simulink model "VehicleDynamics3D"  (R2019b)
settings: Solver=ode15s  StartTime=0.0  StopTime=StopTime  FixedStep=.001  MaxStep=maxStep  RelTol=relTol  AbsTol=absTol  EnableMultiTasking=on
PreLoadFcn:
  | VehicleDynamicsInitialization
model workspace: external: MATLAB File sm_suspension_templates_params.m (data not in the file)
values from neighbouring files (symbols this model uses):
  followerCameraX = 7.5    [VehicleDynamicsInitialization.m]
  followerCameraZ = 3    [VehicleDynamicsInitialization.m]
  frontCameraX = -1.75    [VehicleDynamicsInitialization.m]
  frontCameraZ = 0.35    [VehicleDynamicsInitialization.m]
  isoCameraAimX = (1/2)*wheelbase    (= 0.75)    [VehicleDynamicsInitialization.m]
  isoCameraX = -3.1    [VehicleDynamicsInitialization.m]
  isoCameraY = 3.5    [VehicleDynamicsInitialization.m]
  isoCameraZ = 1.5    [VehicleDynamicsInitialization.m]
  Load = 200    [VehicleDynamicsInitialization.m]
  maxSteeringDisplacement = 10    [VehicleDynamicsInitialization.m]
  minSteeringDisplacement = -10    [VehicleDynamicsInitialization.m]
  SetPaceSampleTime = 0.1    [VehicleDynamicsInitialization.m]
  steeringInput = 0    [VehicleDynamicsInitialization.m]
  vehicleSpeed_kph = 0    [VehicleDynamicsInitialization.m]
  wheelbase = 1.5    [VehicleDynamicsInitialization.m]
undefined symbols (not defined in the file or in its folder): dwb, Floor, sigbuilder_block, wheel, X, Y, Z
libraries: sm_lib x195, sm_suspension_templates_lib x34, nesl_utility x15, Contact_Forces_Lib x4, simulink x2, fl_ps_legacy_lib x1, aerolibanimutils x1
(part 1 of 8)
CloseFcn:
  | clear simlog_sm_suspension_templates
Description:
  | Independent Suspension System Templates
  | 
  | Copyright 2016-2017 The MathWorks, Inc.
settings Model: Creator=MathWorks  LastModifiedBy=adityaaaap
settings SolverCC: AutoScaleAbsTol=off  ZeroCrossAlgorithm=Adaptive
settings DataIOCC: SaveFormat=Array  SaveOutput=off  ReturnWorkspaceOutputsName=FrameCopy_spidata
settings OptimizationCC: ExpressionDepthLimit=2147483647  LifeSpan=inf
settings DebuggingCC: UnderspecifiedInitializationDetection=Classic  MergeDetectMultiDrivingBlocksExec=none  MaskedZcDiagnostic=none  IgnoredZcDiagnostic=none  AllowSymbolicDim=off  StateNameClashWarn=warning  SFUnexpectedBacktrackingDiag=warning  SFNoUnconditionalDefaultTransitionDiag=warning  SFExecutionAtInitializationDiag=none  ArithmeticOperatorsInVariantConditions=warning
settings HardwareCC: ProdBitPerPointer=32  ProdBitPerSizeT=32  ProdBitPerPtrDiffT=32  ProdLargestAtomicFloat=None  ProdIntDivRoundTo=Undefined  ProdEndianess=Unspecified  ProdWordSize=32  ProdHWDeviceType=32-bit Generic
settings ModelReferenceCC: PropagateSignalLabelsOutOfModel=off
settings SFSimCC: SimUseLocalCustomCode=off  SimBuildMode=sf_make  CustomCodeUndefinedFunction=UseInterfaceOnly
settings RTWCC: RTWUseLocalCustomCode=off
settings CodeAppCC: StateflowObjectComments=on
settings GRTTargetCC: TargetLangStandard=C89/C90 (ANSI)  GeneratePreprocessorConditionals=Disable all
settings ConfigComp: CovScope=ReferencedModels  CovIncludeTopModel=off  CovMetricSettings=dw  CovHtmlReporting=on  CovSaveCumulativeToWorkspaceVar=on  CovSaveSingleToWorkspaceVar=on  CovExternalEMLEnable=off  CovSFcnEnable=off
settings SimscapeCC: SimscapeNormalizeSystem=off  SimscapeLogSimulationStatistics=on  SimscapeLogLimitData=off  SimscapeLogDataHistory=10000
settings ConfigurationSet: Description=SimMechanics 2G
settings DiagnosticsConfigSet: SimMechanicsUnconnectedFramePorts=none  SimMechanicsRigidlyBoundBlock=none  SimMechanicsUnsatisfiedHighPriorityTargets=none
settings ExplorerConfigSet: InternalSimMechanicsExplorerSettings="<ExplorerConfiguration><canonicalview>default</canonicalview><AnimationSetting><BasePlaybackSpeed>1.0</BasePlaybackSpeed><PlaybackSpeedFactor>1.0</PlaybackSpeedFactor></AnimationSetting><TilePanel><TileInfo><Tiles Columns=\"2\" Count=\"3\" Rows=\"2\"><Column Left=\"2\" Weight=\"0.4529\"/><Column Left=\"381\" Weight=\"0.5471\"/><Column Left=\"837\"/><Row Top=\"2\" Weight=\"0.5729\"/><Row Top=\"598\" Weight=\"0.4271\"/><Row Top=\"1044\"/><Tile Height=\"2\" Width=\"1\" X=\"0\" Y=\"0\"/><Tile Height=\"1\" Width=\"1\" X=\"1\" Y=\"0\"/><Tile Height=\"1\" Width=\"1\" X=\"1\" Y=\"1\"/></Tiles></TileInfo><SceneInfo><SceneViewer><BGColor><R>0.60000002384185791</R><G>0.60000002384185791</G><B>0.60000002384185791</B></BGColor><Camera><DoPerspective>on</DoPerspective><Position><X>-1.1537063873740901e-15</X><Y>-7.5000000000000018</Y><Z>3.2999999999999994</Z></Position><Center><X>6.6613381477509392e-16</X><Y>1.1102230246251565e-16</Y><Z>0.29999999999999993</Z></Center><Up><X>-5.1501888403816389e-17</X><Y>-7.1161584930853499e-17</Y><Z>1</Z></Up><ViewLimDist>1</ViewLimDist><YLim>0.46630765815499858</YLim><XLim>0.16702210408262291</XLim></Camera></SceneViewer><SceneViewer><BGColor><R>0.60000002384185791</R><G>0.60000002384185791</G><B>0.60000002384185791</B></BGColor><Camera><DoPerspective>on</DoPerspective><Position><X>3.5000000000000018</X><Y>3.0999999999999996</Y><Z>1.8000000000000003</Z></Position><Center><X>4.9960036108132044e-16</X><Y>-0.75000000000000011</Y><Z>0.29999999999999988</Z></Center><Up><X>0</X><Y>0</Y><Z>1</Z></Up><ViewLimDist>1</ViewLimDist><YLim>0.46630765815499858</YLim><XLim>0.35509288448941123</XLim></Camera></SceneViewer><SceneViewer><BGColor><R>0.60000002384185791</R><G>0.60000002384185791</G><B>0.60000002384185791</B></BGColor><Camera><DoPerspective>on</DoPerspective><Position><X>1.036686212452563e-15</X><Y>1.7500000000000004</Y><Z>0.65000000000000002</Z></Position><Center><X>6.6613381477509392e-16</X><Y>1.1102230246251565e-16</Y><Z>0.29999999999999993</Z></Center><Up><X>-5.1501888403816389e-17</X><Y>-7.1161584930853499e-17</Y><Z>1</Z></Up><ViewLimDist>1</ViewLimDist><YLim>0.46630765815499858</YLim><XLim>0.47697831394801909</XLim></Camera></SceneViewer></SceneInfo></TilePanel><MechEditorPanel><Cameras><Camera><Id>Camera1</Id><Value><Name>Follower Camera</Name><NativeCamera><PositionTrackingFeature>Cameras.Follower_Camera_Transform.F</PositionTrackingFeature><CenterTrackingFeature>Cameras.Follower_Camera_Transform.B</CenterTrackingFeature><UpVectorTrackingFeature>Cameras.Follower_Camera_Transform.B</UpVectorTrackingFeature><CenterTrackingOrigin>on</CenterTrackingOrigin><UpVectorTrackingDirection>+Z</UpVectorTrackingDirection></NativeCamera></Value></Camera><Camera><Id>Camera2</Id><Value><Name>Isometric Camera</Name><NativeCamera><PositionTrackingFeature>Cameras.Isometric_Camera_Transform.F</PositionTrackingFeature><CenterTrackingFeature>Cameras.Isometric_Camera_Aim.F</CenterTrackingFeature><UpVectorTrackingFeature>Floor_And_Grid.World_Frame.W</UpVectorTrackingFeature><CenterTrackingOrigin>on</CenterTrackingOrigin><UpVectorTrackingDirection>+Z</UpVectorTrackingDirection></NativeCamera></Value></Camera><Camera><Id>Camera3</Id><Value><Name>Front Camera</Name><NativeCamera><PositionTrackingFeature>Cameras.Front_Camera_Transform.F</PositionTrackingFeature><CenterTrackingFeature>Cameras.Front_Camera_Transform.B</CenterTrackingFeature><UpVectorTrackingFeature>Cameras.Front_Camera_Transform.B</UpVectorTrackingFeature><CenterTrackingOrigin>on</CenterTrackingOrigin><UpVectorTrackingDirection>+Z</UpVectorTrackingDirection></NativeCamera></Value></Camera></Cameras><GfxPanelCameraMap><MapElement CameraMLId=\"Camera1\" GfxPanelIndex=\"0\"/><MapElement CameraMLId=\"Camera2\" GfxPanelIndex=\"1\"/><MapElement CameraMLId=\"Camera3\" GfxPanelIndex=\"2\"/></GfxPanelCameraMap><VideoCreator><PlaybackSpeedRatio>1.0</PlaybackSpeedRatio><FrameRate>30</FrameRate><VideoFormat>Motion JPEG AVI</VideoFormat><FrameSize>auto</FrameSize></VideoCreator></MechEditorPanel></ExplorerConfiguration>"

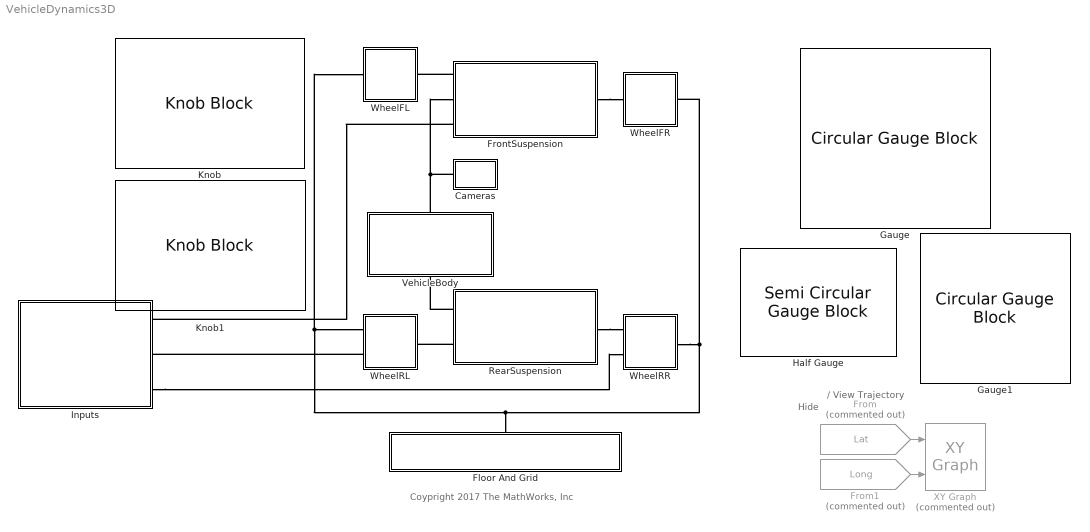
== system VehicleDynamics3D ==
  note: Hide
  note: / View Trajectory
  note: Coypright 2017 The MathWorks, Inc
  Cameras : Subsystem
      mask Display: image('CameraPic.png');
  Floor And Grid : Subsystem
      mask Display: image('Floor.png');
  From : From  Commented=on  GotoTag=Lat  TagVisibility=global
  From1 : From  Commented=on  GotoTag=Long  TagVisibility=global
  FrontSuspension : Subsystem  VariantControl=DoubleWishbone
      mask Display:
      | image(imread(fullfile(matlabroot,...
      |     'toolbox','physmod','sm','smdemos',...
      |     'suspension_templates','images','sm_isuspension_dwishbone.png')));
  Gauge : CircularGaugeBlock  ScaleMax=50
  Gauge1 : CircularGaugeBlock  ScaleMin=-180  ScaleMax=180  TickInterval=45
  Half Gauge : SemiCircularGaugeBlock  ScaleMin=-1  ScaleMax=1  TickInterval=0.5
  Inputs : Subsystem  mask(User Input){UserOption=Slalom}
      mask prompts: UserOption "User Input Mode"
      mask help: Choose the input to the vehicle. Input can be a driving maneuver or manual driving.
      mask TypeOptions UserOption: Slalom | Right Turn 90° | Left Turn 90° | Steep Steer | Burnout | Skidpad | Dashboard Instruments
      mask Callback UserOption:
      | StopTime = 15;
      | relTol = 1E-4;
      | absTol = 1E-5;
      | maxStep = 1E-2;
      | 
      | currvalue = get_param([bdroot '/Inputs'],'UserOption');
      | if isequal(currvalue,'Slalom')
      |     UserInput = 1;
      |     graphXMin = -10;
      |     graphXMax = 10;
      |     graphYmin = 0;
      |     graphYMax = 120;
      | elseif isequal(currvalue,'Right Turn 90°')
      |     UserInput = 2;
      |     graphXMin = -50;
      |     graphXMax = 50;
      |     graphYmin = 0;
      |     graphYMax = 50;
      |  elseif isequal(currvalue,'Left Turn 90°')
      |     UserInput = 3;
      |     graphXMin = -50;
      |     graphXMax = 50;
      |     graphYmin = 0;
      |     graphYMax = 50;
      | elseif isequal(currvalue,'Steep Steer')
      |     UserInput = 4;
      |     graphXMin = -70;
      |     graphXMax = 70;
      |     graphYmin = -70;
      |     graphYMax = 70;
      | elseif isequal(currvalue,'Burnout')
      |     UserInput = 5;
      |     graphXMin = -20;
      |     graphXMax = 20;
      |     graphYmin = -10;
      |     graphYMax = 10;
      | elseif isequal(currvalue,'Skidpad')
      |     UserInput = 6;
      |     StopTime = 40;
      |     graphXMin = -30;
      |     graphXMax = 30;
      |     graphYmin = -30;
      |     graphYMax = 30;
      | else
      |     UserInput = 7;
      |     StopTime = inf;
      |     relTol = 1E-1;
      |     absTol = 1E-2;
      |     maxStep = 0.2;
      |     graphXMin = -500;
      |     graphXMax = 500;
      |     graphYmin = -500;
      |     graphYMax = 500;
      | end
      mask Display:
      | currvalue = get_param([bdroot '/Inputs'],'UserOption');
      | if isequal(currvalue,'Slalom')
      |     image('SlalomPic.png')
      | elseif isequal(currvalue,'Right Turn 90°')
      |     image('RightTurnPic.png')
      | elseif isequal(currvalue,'Left Turn 90°')
      |     image('LeftTurnPic.png')
      | elseif isequal(currvalue,'Steep Steer')
      |     image('SteepSteerPic.png')
      | elseif isequal(currvalue,'Burnout')
      |     image('BurnoutPic.png')
      | elseif isequal(currvalue,'Skidpad')
      |     image('SkidpadPic.png')
      | else
      |     image('DashboardPic.png')
      | end
      | 
      | port_label('RConn',1,'S');
      | port_label('RConn',2,'L');
      | port_label('RConn',3,'R');
  Knob : KnobBlock  ScaleMin=-10  ScaleMax=10  TickInterval=2
  Knob1 : KnobBlock  ScaleMax=50  TickInterval=5
  RearSuspension : Subsystem  VariantControl=DoubleWishbone
      mask Display:
      | image(imread(fullfile(matlabroot,...
      |     'toolbox','physmod','sm','smdemos',...
      |     'suspension_templates','images','sm_isuspension_dwishbone.png')));
  VehicleBody : Subsystem
      mask Display: image('VehicleBodyPic.png');
  WheelFL : Subsystem  mask(Wheel){Rti=wheel.tire.innerradius, Rto=wheel.tire.outerradius, Wt=wheel.tire.width, Rtr=wheel.tire.chamferradius, trho=wheel.tire.density, tclr=wheel.tire.color, Rhi=wheel.hub.radius, Rho=wheel.hub.outerradius, Ns=wheel.hub.numspokes, Ts=wheel.hub.spokethickness, Wh=wheel.hub.width, srho=wheel.hub.density, sclr=wheel.hub.color, Ls=wheel.shaft.length, Rs=wheel.shaft.radius, Rb=wheel.disc.radius, Tb=wheel.disc.thickness}
      mask prompts: Rti "Tire inner radius (cm):"; Rto "Tire outer radius (cm):"; Wt "Tire width (cm):"; Rtr "Chamfer/fillet radius (cm):"; trho "Density (kg/m^3):"; tclr "Color ([r  g b]):"; Rhi "Hub radius (cm):"; Rho "Outer radius of spokes (cm):"; Ns "Number of spokes:"; Ts "Thickness of spokes:"; Wh "Width of hub (cm):"; srho "Density (kg/m^3):"; sclr "Color ([r g b]):"; Ls "Shaft length (cm):"; Rs "Shaft radius (cm):"; Rb "Brake disc radius (cm):"; Tb "Brake disc thickness (cm):"
      mask help: This block models a wheel assembly. The port H corresponds to the center of the wheel hub. Port T corresponds to the bottom of the tire.
      mask init:
      | spk_angles = linspace(0,2*pi,Ns+1);
      | 
      | spokes_xsec = [];
      | r_indices = [];
      | wang = 20*pi/180;
      | for idx = 1:length(spk_angles)-1
      |     ang = spk_angles(idx);
      |     theta = linspace(ang-wang,ang+wang,20)';
      |     spokes_xsec = [spokes_xsec;
      |                    Rhi*cos(theta) Rhi*sin(theta)];
      |     theta = linspace(ang+wang, spk_angles(idx+1)-wang, 50)';
      |     len = length(spokes_xsec);
      |     r_indices = [r_indices len len+1];
      |     spokes_xsec = [spokes_xsec;
      |                    Rho*cos(theta) Rho*sin(theta)];
      | end
      | 
      | rim_xsec = [Rho -Wh/2; Rti -Wt/2; 
      |             Rti Wt/2; Rho Wh/2+Ts];
      | 
      | tire_xsec = [Rti -Wt/2; Rto -Wt/2; Rto Wt/2; Rti Wt/2];
      | tire_xsec = simmechanics.demohelpers.round_corners(tire_xsec,1:4,Rtr,10);
      mask DialogControl ParameterTabVar0 Prompt: Tire
      mask DialogControl ParameterTabVar01 Prompt: Hub
      mask DialogControl ParameterTabVar012 Prompt: Brake and Shaft
      mask Display:
      | image(imread(fullfile(matlabroot,...
      |     'toolbox','physmod','sm','smdemos',...
      |     'suspension_templates','images','sm_isuspension_wheel.png')));
      | 
      | port_label('LConn',1,'H');
      | port_label('RConn',1,'T');
  WheelFR : Subsystem  mask(Wheel){Rti=wheel.tire.innerradius, Rto=wheel.tire.outerradius, Wt=wheel.tire.width, Rtr=wheel.tire.chamferradius, trho=wheel.tire.density, tclr=wheel.tire.color, Rhi=wheel.hub.radius, Rho=wheel.hub.outerradius, Ns=wheel.hub.numspokes, Ts=wheel.hub.spokethickness, Wh=wheel.hub.width, srho=wheel.hub.density, sclr=wheel.hub.color, Ls=wheel.shaft.length, Rs=wheel.shaft.radius, Rb=wheel.disc.radius, Tb=wheel.disc.thickness}
      mask prompts: Rti "Tire inner radius (cm):"; Rto "Tire outer radius (cm):"; Wt "Tire width (cm):"; Rtr "Chamfer/fillet radius (cm):"; trho "Density (kg/m^3):"; tclr "Color ([r  g b]):"; Rhi "Hub radius (cm):"; Rho "Outer radius of spokes (cm):"; Ns "Number of spokes:"; Ts "Thickness of spokes:"; Wh "Width of hub (cm):"; srho "Density (kg/m^3):"; sclr "Color ([r g b]):"; Ls "Shaft length (cm):"; Rs "Shaft radius (cm):"; Rb "Brake disc radius (cm):"; Tb "Brake disc thickness (cm):"
      mask help: This block models a wheel assembly. The port H corresponds to the center of the wheel hub. Port T corresponds to the bottom of the tire.
      mask init: same as VehicleDynamics3D/WheelFL
      mask DialogControl ParameterTabVar0 Prompt: Tire
      mask DialogControl ParameterTabVar01 Prompt: Hub
      mask DialogControl ParameterTabVar012 Prompt: Brake and Shaft
      mask Display:
      | image(imread(fullfile(matlabroot,...
      |     'toolbox','physmod','sm','smdemos',...
      |     'suspension_templates','images','sm_isuspension_wheel.png')));
      | 
      | port_label('LConn',1,'H');
      | port_label('RConn',1,'T');
  WheelRL : Subsystem  mask(Wheel){Rti=wheel.tire.innerradius, Rto=wheel.tire.outerradius, Wt=wheel.tire.width, Rtr=wheel.tire.chamferradius, trho=wheel.tire.density, tclr=wheel.tire.color, Rhi=wheel.hub.radius, Rho=wheel.hub.outerradius, Ns=wheel.hub.numspokes, Ts=wheel.hub.spokethickness, Wh=wheel.hub.width, srho=wheel.hub.density, sclr=wheel.hub.color, Ls=wheel.shaft.length, Rs=wheel.shaft.radius, Rb=wheel.disc.radius, Tb=wheel.disc.thickness}
      mask prompts: Rti "Tire inner radius (cm):"; Rto "Tire outer radius (cm):"; Wt "Tire width (cm):"; Rtr "Chamfer/fillet radius (cm):"; trho "Density (kg/m^3):"; tclr "Color ([r  g b]):"; Rhi "Hub radius (cm):"; Rho "Outer radius of spokes (cm):"; Ns "Number of spokes:"; Ts "Thickness of spokes:"; Wh "Width of hub (cm):"; srho "Density (kg/m^3):"; sclr "Color ([r g b]):"; Ls "Shaft length (cm):"; Rs "Shaft radius (cm):"; Rb "Brake disc radius (cm):"; Tb "Brake disc thickness (cm):"
      mask help: This block models a wheel assembly. The port H corresponds to the center of the wheel hub. Port T corresponds to the bottom of the tire.
      mask init: same as VehicleDynamics3D/WheelFL
      mask DialogControl ParameterTabVar0 Prompt: Tire
      mask DialogControl ParameterTabVar01 Prompt: Hub
      mask DialogControl ParameterTabVar012 Prompt: Brake and Shaft
      mask Display:
      | image(imread(fullfile(matlabroot,...
      |     'toolbox','physmod','sm','smdemos',...
      |     'suspension_templates','images','sm_isuspension_wheel.png')));
      | 
      | port_label('LConn',1,'H');
      | port_label('RConn',1,'T');
  WheelRR : Subsystem  mask(Wheel){Rti=wheel.tire.innerradius, Rto=wheel.tire.outerradius, Wt=wheel.tire.width, Rtr=wheel.tire.chamferradius, trho=wheel.tire.density, tclr=wheel.tire.color, Rhi=wheel.hub.radius, Rho=wheel.hub.outerradius, Ns=wheel.hub.numspokes, Ts=wheel.hub.spokethickness, Wh=wheel.hub.width, srho=wheel.hub.density, sclr=wheel.hub.color, Ls=wheel.shaft.length, Rs=wheel.shaft.radius, Rb=wheel.disc.radius, Tb=wheel.disc.thickness}
      mask prompts: Rti "Tire inner radius (cm):"; Rto "Tire outer radius (cm):"; Wt "Tire width (cm):"; Rtr "Chamfer/fillet radius (cm):"; trho "Density (kg/m^3):"; tclr "Color ([r  g b]):"; Rhi "Hub radius (cm):"; Rho "Outer radius of spokes (cm):"; Ns "Number of spokes:"; Ts "Thickness of spokes:"; Wh "Width of hub (cm):"; srho "Density (kg/m^3):"; sclr "Color ([r g b]):"; Ls "Shaft length (cm):"; Rs "Shaft radius (cm):"; Rb "Brake disc radius (cm):"; Tb "Brake disc thickness (cm):"
      mask help: This block models a wheel assembly. The port H corresponds to the center of the wheel hub. Port T corresponds to the bottom of the tire.
      mask init: same as VehicleDynamics3D/WheelFL
      mask DialogControl ParameterTabVar0 Prompt: Tire
      mask DialogControl ParameterTabVar01 Prompt: Hub
      mask DialogControl ParameterTabVar012 Prompt: Brake and Shaft
      mask Display:
      | image(imread(fullfile(matlabroot,...
      |     'toolbox','physmod','sm','smdemos',...
      |     'suspension_templates','images','sm_isuspension_wheel.png')));
      | 
      | port_label('LConn',1,'H');
      | port_label('RConn',1,'T');
  XY Graph : simulink/Sinks/XY Graph  Commented=on  xmin=graphXMin  xmax=graphXMax  ymin=graphYmin  ymax=graphYMax  st=0.5
  wires:
  From/1 -> XY Graph/1
  From1/1 -> XY Graph/2
  connections:
  FrontSuspension/LConn1 -- WheelFL/LConn1
  FrontSuspension/RConn1 -- WheelFR/LConn1
  RearSuspension/RConn1 -- WheelRR/LConn1
  WheelRL/RConn1 -- WheelFL/RConn1 -- WheelRR/RConn1 -- WheelFR/RConn1 -- Floor And Grid/RConn1
  RearSuspension/LConn2 -- WheelRL/LConn1
  Cameras/LConn1 -- VehicleBody/LConn1 -- FrontSuspension/LConn2
  RearSuspension/LConn1 -- VehicleBody/RConn1
  WheelRL/RConn2 -- Inputs/RConn2
  Inputs/RConn3 -- WheelRR/LConn2
  FrontSuspension/LConn3 -- Inputs/RConn1

== system VehicleDynamics3D/Cameras ==
  Follower Camera Transform : sm_lib/Frames and Transforms/Rigid Transform  TranslationMethod=Cartesian  TranslationStandardOffset=0  TranslationLengthUnit=m  TranslationStandardAxis=+Z  TranslationCartesianOffset=[followerCameraX 0 followerCameraZ ]  TranslationROffset=0  TranslationROffsetUnits=m  TranslationZOffset=0  TranslationZOffsetUnits=m  TranslationThetaOffset=0  TranslationThetaOffsetUnits=deg  RotationMethod=None  RotationAngleUnits=deg  RotationStandardAxis=+Z  RotationAngle=0.0  RotationArbitraryAxis=[0 0 1]  FollAlignAxisA=+X  BaseAlignAxisA=+Y  FollAlignAxisB=+Y  BaseAlignAxisB=+Z  RotationSequenceAxes=FollowerAxes  RotationSequence=XYX  RotationSequenceAngles=[0 0 0]  RotationSequenceAnglesUnits=deg  RotationMatrix=[1 0 0; 0 1 0; 0 0 1]
  Front Camera Transform : sm_lib/Frames and Transforms/Rigid Transform  TranslationMethod=Cartesian  TranslationStandardOffset=0  TranslationLengthUnit=m  TranslationStandardAxis=+Z  TranslationCartesianOffset=[frontCameraX 0 frontCameraZ]  TranslationROffset=0  TranslationROffsetUnits=m  TranslationZOffset=0  TranslationZOffsetUnits=m  TranslationThetaOffset=0  TranslationThetaOffsetUnits=deg  RotationMethod=None  RotationAngleUnits=deg  RotationStandardAxis=+Z  RotationAngle=0.0  RotationArbitraryAxis=[0 0 1]  FollAlignAxisA=+X  BaseAlignAxisA=+Y  FollAlignAxisB=+Y  BaseAlignAxisB=+Z  RotationSequenceAxes=FollowerAxes  RotationSequence=XYX  RotationSequenceAngles=[0 0 0]  RotationSequenceAnglesUnits=deg  RotationMatrix=[1 0 0; 0 1 0; 0 0 1]
  Isometric Camera Transform : sm_lib/Frames and Transforms/Rigid Transform  TranslationMethod=Cartesian  TranslationStandardOffset=0  TranslationLengthUnit=m  TranslationStandardAxis=+Z  TranslationCartesianOffset=[isoCameraX isoCameraY isoCameraZ]  TranslationROffset=0  TranslationROffsetUnits=m  TranslationZOffset=0  TranslationZOffsetUnits=m  TranslationThetaOffset=0  TranslationThetaOffsetUnits=deg  RotationMethod=None  RotationAngleUnits=deg  RotationStandardAxis=+Z  RotationAngle=0.0  RotationArbitraryAxis=[0 0 1]  FollAlignAxisA=+X  BaseAlignAxisA=+Y  FollAlignAxisB=+Y  BaseAlignAxisB=+Z  RotationSequenceAxes=FollowerAxes  RotationSequence=XYX  RotationSequenceAngles=[0 0 0]  RotationSequenceAnglesUnits=deg  RotationMatrix=[1 0 0; 0 1 0; 0 0 1]
  Isometric Camera Aim : sm_lib/Frames and Transforms/Rigid Transform  TranslationMethod=Cartesian  TranslationStandardOffset=0  TranslationLengthUnit=m  TranslationStandardAxis=+Z  TranslationCartesianOffset=[isoCameraAimX 0 0]  TranslationROffset=0  TranslationROffsetUnits=m  TranslationZOffset=0  TranslationZOffsetUnits=m  TranslationThetaOffset=0  TranslationThetaOffsetUnits=deg  RotationMethod=None  RotationAngleUnits=deg  RotationStandardAxis=+Z  RotationAngle=0.0  RotationArbitraryAxis=[0 0 1]  FollAlignAxisA=+X  BaseAlignAxisA=+Y  FollAlignAxisB=+Y  BaseAlignAxisB=+Z  RotationSequenceAxes=FollowerAxes  RotationSequence=XYX  RotationSequenceAngles=[0 0 0]  RotationSequenceAnglesUnits=deg  RotationMatrix=[1 0 0; 0 1 0; 0 0 1]
  PS Integrator : fl_ps_legacy_lib/Legacy Physical Signals/Linear Operators/PS Integrator  x0=0
      settings: SourceProductName=Simscape  SourceProductBaseCode=SS  InternalSimscapePortConfiguration="{\"Bottom\":[],\"Left\":[{\"id\":\"I\",\"label\":\"\",\"type\":\"input\"}],\"Right\":[{\"id\":\"O\",\"label\":\"\",\"type\":\"output\"}],\"Top\":[]}"
  Revolute Joint : sm_lib/Joints/Revolute Joint  JointMode=Normal  SenseConstraintForce=off  SenseConstraintForceX=off  SenseConstraintForceY=off  SenseConstraintForceZ=off  SenseConstraintTorque=off  SenseConstraintTorqueX=off  SenseConstraintTorqueY=off  SenseConstraintTorqueZ=off  SenseTotalForce=off  SenseTotalForceX=off  SenseTotalForceY=off  SenseTotalForceZ=off  SenseTotalTorque=off  SenseTotalTorqueX=off  SenseTotalTorqueY=off  SenseTotalTorqueZ=off  CompositeWrenchDir=FollowerOnBase  CompositeWrenchFrame=BaseFrame  EquilibriumPosition=0  EquilibriumPositionUnits=deg  SpringStiffness=IsoCameraStiffness  SpringStiffnessUnits=N*m/deg  DampingCoefficient=IsoCameraDamping  DampingCoefficientUnits=N*m/(deg/s)  TorqueActuationMode=ComputedTorque  MotionActuationMode=InputMotion  SensePosition=off  SenseVelocity=off  SenseAcceleration=off  SenseTorqueForce=off  SenseLowerLimitTorqueForce=off  SenseUpperLimitTorqueForce=off  LowerLimitSpecify=off  LowerLimitBound=-90  LowerLimitBoundUnits=deg  LowerLimitStiffness=1e4  LowerLimitStiffnessUnits=N*m/deg  LowerLimitDamping=10  LowerLimitDampingUnits=N*m/(deg/s)  LowerLimitTransitionRegionWidth=0.1  LowerLimitTransitionRegionWidthUnits=deg  UpperLimitSpecify=off  UpperLimitBound=90  UpperLimitBoundUnits=deg  UpperLimitStiffness=1e4  UpperLimitStiffnessUnits=N*m/deg  UpperLimitDamping=10  UpperLimitDampingUnits=N*m/(deg/s)  UpperLimitTransitionRegionWidth=0.1  UpperLimitTransitionRegionWidthUnits=deg  PositionTargetSpecify=off  PositionTargetPriority=High  PositionTargetValue=0  PositionTargetValueUnits=deg  VelocityTargetSpecify=off  VelocityTargetPriority=High  VelocityTargetValue=0  VelocityTargetValueUnits=deg/s
  Solid : sm_lib/Body Elements/Brick Solid  GraphicAmbientColor=[0.15 0.15 0.15 1.0]  BasedOnType=Density  BrickDimensions=[1 1 1]  BrickDimensionUnits=mm  CenterOfMass=[0 0 0]  CenterOfMassUnits=m  GraphicDiffuseColor=[0.5 0.5 0.5]  Density=1000  DensityUnits=kg/m^3  DoExposeReferenceFrame=on  GraphicEmissiveColor=[0.0 0.0 0.0 1.0]  ExportEntireGeometry=off  SerializedFrames=<Frames/>  MarkerShape=Sphere  MarkerSize=10  GraphicType=FromGeometry  InertiaType=PointMass  Mass=1E-03  MassUnits=kg  MomentsOfInertia=[1 1 1]  MomentsOfInertiaUnits=kg*m^2  GraphicOpacity=0  ProductsOfInertia=[1 1 1]  ProductsOfInertiaUnits=kg*m^2  GraphicShininess=75  GraphicSpecularColor=[0.5 0.5 0.5 1.0]  GraphicVisPropType=SimpleVisualProperties
  Transform Sensor : sm_lib/Frames and Transforms/Transform Sensor  MeasurementFrame=Base  SenseAngle=off  SenseAxis=off  SenseAngle1=off  SenseAngle2=off  SenseAngle3=off  SenseQ=off  SenseR=off  SenseOmegaX=off  SenseOmegaY=off  SenseOmegaZ=on  SenseOmega1=off  SenseOmega2=off  SenseOmega3=off  SenseQDot=off  SenseRDot=off  SenseAlphaX=off  SenseAlphaY=off  SenseAlphaZ=off  SenseAlpha1=off  SenseAlpha2=off  SenseAlpha3=off  SenseQDDot=off  SenseRDDot=off  SenseX=off  SenseY=off  SenseZ=off  SenseRad=off  SenseAzim=off  SenseDist=off  SenseInc=off  SenseXDot=off  SenseYDot=off  SenseZDot=off  SenseRadDot=off  SenseAzimDot=off  SenseDistDot=off  SenseIncDot=off  SenseXDDot=off  SenseYDDot=off  SenseZDDot=off  SenseRadDDot=off  SenseAzimDDot=off  SenseDistDDot=off  SenseIncDDot=off
  " " : PMIOPort  Side=Left
  connections:
  Follower Camera Transform/LConn1 -- Isometric Camera Aim/LConn1 -- Revolute Joint/LConn1 -- Transform Sensor/LConn1 -- Front Camera Transform/LConn1 -- " "/RConn1
  Revolute Joint/RConn1 -- Solid/RConn1 -- Isometric Camera Transform/LConn1
  Transform Sensor/RConn2 -- PS Integrator/LConn1
  PS Integrator/RConn1 -- Revolute Joint/LConn2

== system VehicleDynamics3D/Floor And Grid ==
  Floor : sm_lib/Body Elements/Brick Solid  GraphicAmbientColor=[0.15 0.15 0.15 1.0]  BasedOnType=Density  BrickDimensions=[Floor.l , Floor.w , Floor.h]  BrickDimensionUnits=m  CenterOfMass=[0 0 0]  CenterOfMassUnits=m  GraphicDiffuseColor=[0.6 0.6 0.6]  Density=1000  DensityUnits=kg/(m^3)  DoExposeReferenceFrame=on  GraphicEmissiveColor=[0.0 0.0 0.0 1.0]  ExportEntireGeometry=off  SerializedFrames=<Frames/>  MarkerShape=Sphere  MarkerSize=10  GraphicType=FromGeometry  InertiaType=CalculateFromGeometry  Mass=1  MassUnits=kg  MomentsOfInertia=[1 1 1]  MomentsOfInertiaUnits=kg*m^2  GraphicOpacity=1.0  ProductsOfInertia=[0 0 0]  ProductsOfInertiaUnits=kg*m^2  GraphicShininess=75  GraphicSpecularColor=[0.5 0.5 0.5 1.0]  GraphicVisPropType=AdvancedVisualProperties
  Grid : Subsystem
  Mechanism Configuration : sm_lib/Utilities/Mechanism Configuration  UniformGravity=Constant  GravityVector=[0 0 -9.80665]  GravityUnits=m/s^2  LinearizationDelta=0.001
  Solver Configuration : nesl_utility/Solver Configuration  PhysicalDomain=network_engine_domain  SubClassName=solver  LeftPortType=input  RightPortType=generic  Tones=[]  Harmonics=[]  SimulateNoise=off  Profile=off  UseLocalSampling=off  EnableSwitchedLinearOptims=on  FrequencyDomain=off  UseCCode=off  RelTol=0.001  AbsTol=1e-06  MinStep=1e-09  ToWorkspace=off  RevertToSquareIcSolve=off  NumHomotopyIterations=100  PhasorMode=off  PhasorModeNumHarmonics=1  DoDC=off  ResidualTolerance=1e-09  UseLocalSolver=off  LocalSolverChoice=NE_BACKWARD_EULER_ADVANCER  LocalSolverSampleTime=0.01  DoFixedCost=off  MaxNonlinIter=3  MaxModeIter=2  LinearAlgebra=Sparse  EquationFormulation=NE_TIME_EF  DelaysMemoryBudget=1024  AutomaticFiltering=on  FilteringTimeConstant=Filtering1Dto3DConnection  PartitionStorageMethod=AS_NEEDED  PartitionMemoryBudget=1024  PartitionMethod=FAST
  World Frame : sm_lib/Frames and Transforms/World Frame
  R : PMIOPort  Side=Right
  connections:
  R/RConn1 -- Mechanism Configuration/RConn1 -- World Frame/RConn1 -- Solver Configuration/RConn1 -- Floor/RConn1 -- Grid/LConn1
